simulink model "plant_2015B"  (R2015b)
settings: Solver=ode1  StartTime=0.0  StopTime=sim_time  FixedStep=0.001  RelTol=1e-3
undefined symbols (not defined in the file): Standard_Devices, UDP_Protocol, zh_step
libraries: sldrtlib x6, dspnetwork x2, powerlib_meascontrol x1
settings Model: Creator=Anony  LastModifiedBy=Anony

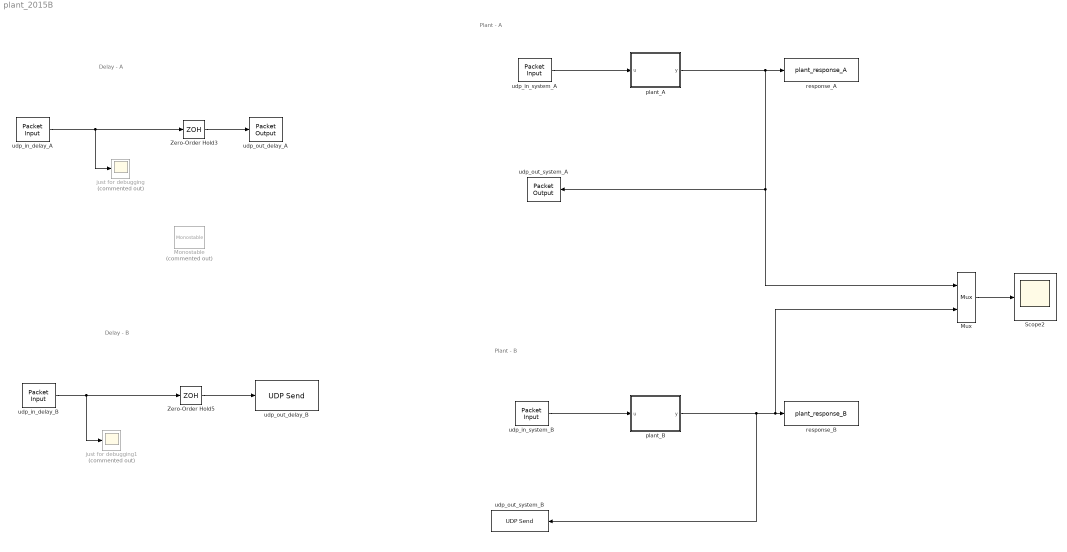
== system plant_2015B ==
  note: Plant - A
  note: Plant - B
  note: Delay - A
  note: Delay - B
  Monostable : powerlib_meascontrol/Logic/Monostable  Commented=on  EdgeDetect=Rising  PulseDuration=0.015  ic=0  Ts=0
  Mux : Mux  Inputs=2
  Scope2 : Scope
  Zero-Order Hold3 : ZeroOrderHold  SampleTime=zh_step
  Zero-Order Hold5 : ZeroOrderHold  SampleTime=zh_step
  just for debugging : Scope  Commented=on
  just for debugging1 : Scope  Commented=on
  plant_A : Subsystem
  plant_B : Subsystem
  response_A : ToWorkspace  VariableName=plant_response_A  SaveFormat=Timeseries  SampleTime=zh_step
  response_B : ToWorkspace  VariableName=plant_response_B  SaveFormat=Timeseries  SampleTime=zh_step
  udp_in_delay_A : sldrtlib/Packet Input  SampleTime=0.001  MaxMissedTicks=inf  ShowMissedTicks=off  YieldWhenWaiting=off  DrvName=Standard_Devices/UDP_Protocol  DrvAddress=27000  DrvOptions=[2468394754 27000]  PacketSize=8  DataTypes='double'  ShowReady=off  ShowError=off  PacketID=1  ByteOrder=1  ShowTimestamp=off
      settings: AttributesFormatString=Standard Devices\nUDP Protocol [6978h]
  udp_in_delay_B : sldrtlib/Packet Input  SampleTime=0.001  MaxMissedTicks=inf  ShowMissedTicks=off  YieldWhenWaiting=off  DrvName=Standard_Devices/UDP_Protocol  DrvAddress=27010  DrvOptions=[2468394754 27010]  PacketSize=8  DataTypes='double'  ShowReady=off  ShowError=off  PacketID=1  ByteOrder=1  ShowTimestamp=off
      settings: AttributesFormatString=Standard Devices\nUDP Protocol [6982h]
  udp_in_system_A : sldrtlib/Packet Input  SampleTime=0.001  MaxMissedTicks=inf  ShowMissedTicks=off  YieldWhenWaiting=off  DrvName=Standard_Devices/UDP_Protocol  DrvAddress=27500  DrvOptions=[2468394754 27500]  PacketSize=8  DataTypes='double'  ShowReady=off  ShowError=off  PacketID=1  ByteOrder=1  ShowTimestamp=off
      settings: AttributesFormatString=Standard Devices\nUDP Protocol [6B6Ch]
  udp_in_system_B : sldrtlib/Packet Input  SampleTime=0.001  MaxMissedTicks=inf  ShowMissedTicks=off  YieldWhenWaiting=off  DrvName=Standard_Devices/UDP_Protocol  DrvAddress=27510  DrvOptions=[2468394754 27510]  PacketSize=8  DataTypes='double'  ShowReady=off  ShowError=off  PacketID=1  ByteOrder=1  ShowTimestamp=off
      settings: AttributesFormatString=Standard Devices\nUDP Protocol [6B76h]
  udp_out_delay_A : sldrtlib/Packet Output  SampleTime=0.01  MaxMissedTicks=inf  ShowMissedTicks=off  YieldWhenWaiting=off  DrvName=Standard_Devices/UDP_Protocol  DrvAddress=28000  DrvOptions=[2468394754 28000]  PacketSize=8  DataTypes='double'  ShowReady=off  ShowError=off  PacketID=1  ByteOrder=1  InitialValue=[]  FinalValue=[]
      settings: AttributesFormatString=Standard Devices\nUDP Protocol [6D60h]
  udp_out_delay_B : dspnetwork/UDP Send  remoteURL='147.32.183.2'  remotePort=28010  localURL='0.0.0.0'  localPortSource=Automatically determine  localPort=27000  sampletime=-1  separateLengthPort=0
  udp_out_system_A : sldrtlib/Packet Output  SampleTime=0.01  MaxMissedTicks=inf  ShowMissedTicks=off  YieldWhenWaiting=off  DrvName=Standard_Devices/UDP_Protocol  DrvAddress=28500  DrvOptions=[2468394754 28500]  PacketSize=8  DataTypes='double'  ShowReady=off  ShowError=off  PacketID=1  ByteOrder=1  InitialValue=[]  FinalValue=[]
      settings: AttributesFormatString=Standard Devices\nUDP Protocol [6F54h]
  udp_out_system_B : dspnetwork/UDP Send  remoteURL='147.32.183.2'  remotePort=28510  localURL='0.0.0.0'  localPortSource=Automatically determine  localPort=27000  sampletime=-1  separateLengthPort=0
  wires:
  plant_A/1(y) -> response_A/1, udp_out_system_A/1, Mux/1
  udp_in_system_A/1 -> plant_A/1(u)
  udp_in_system_B/1 -> plant_B/1(u)
  plant_B/1(y) -> Mux/2, response_B/1, udp_out_system_B/1
  udp_in_delay_A/1 -> just for debugging/1, Zero-Order Hold3/1
  Zero-Order Hold3/1 -> udp_out_delay_A/1
  udp_in_delay_B/1 -> just for debugging1/1, Zero-Order Hold5/1
  Zero-Order Hold5/1 -> udp_out_delay_B/1
  Mux/1 -> Scope2/1

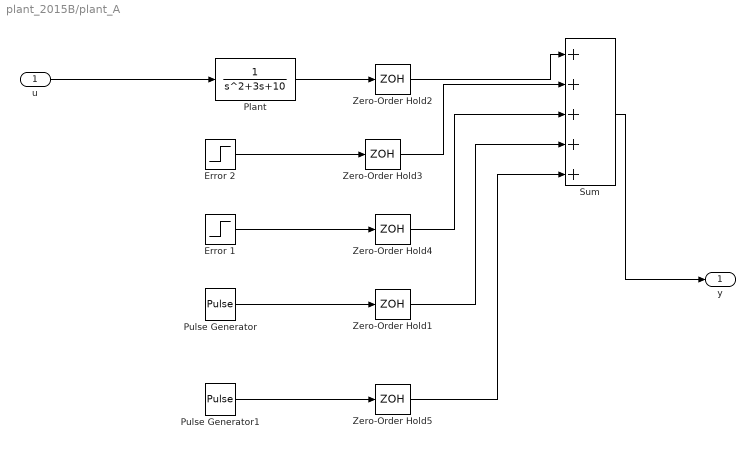
== system plant_2015B/plant_A ==
  u : Inport
  Error 1 : Step  Time=40  After=-0.4  SampleTime=0
  Error 2 : Step  Time=20  After=0.2  SampleTime=0
  Plant : TransferFcn  Denominator=[1 3 10]
  Pulse Generator : DiscretePulseGenerator  PulseType=Time based  Amplitude=0.3  Period=3  PulseWidth=5  PhaseDelay=15
  Pulse Generator1 : DiscretePulseGenerator  PulseType=Time based  Amplitude=-0.18  Period=3  PulseWidth=5  PhaseDelay=25
  Sum : Sum  Inputs=|+++++
  Zero-Order Hold{1..5} (5 alike) : ZeroOrderHold  SampleTime=zh_step
  y : Outport
  wires:
  Zero-Order Hold3/1 -> Sum/2
  Plant/1 -> Zero-Order Hold2/1
  Sum/1 -> y/1
  Zero-Order Hold2/1 -> Sum/1
  u/1 -> Plant/1
  Zero-Order Hold4/1 -> Sum/3
  Error 2/1 -> Zero-Order Hold3/1
  Error 1/1 -> Zero-Order Hold4/1
  Pulse Generator/1 -> Zero-Order Hold1/1
  Zero-Order Hold1/1 -> Sum/4
  Pulse Generator1/1 -> Zero-Order Hold5/1
  Zero-Order Hold5/1 -> Sum/5

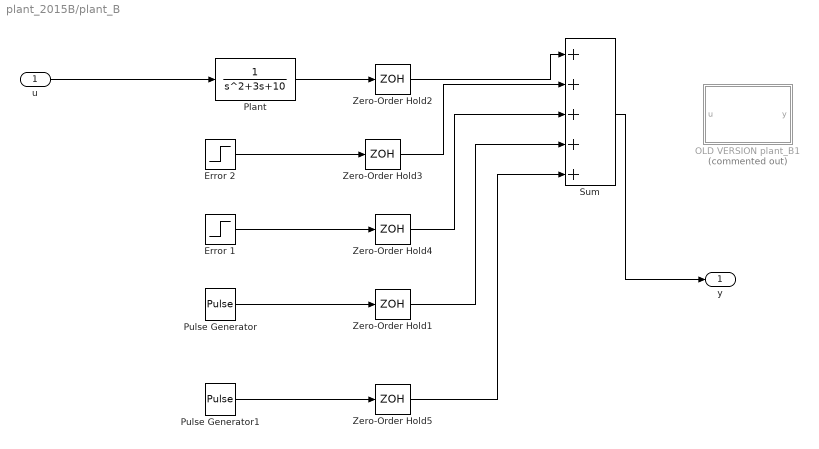
== system plant_2015B/plant_B ==
  u : Inport
  Error 1 : Step  Time=40  After=-0.4  SampleTime=0
  Error 2 : Step  Time=20  After=0.2  SampleTime=0
  OLD VERSION plant_B1 : Subsystem  Commented=on
  Plant : TransferFcn  Denominator=[1 3 10]
  Pulse Generator : DiscretePulseGenerator  PulseType=Time based  Amplitude=0.3  Period=3  PulseWidth=5  PhaseDelay=15
  Pulse Generator1 : DiscretePulseGenerator  PulseType=Time based  Amplitude=-0.18  Period=3  PulseWidth=5  PhaseDelay=25
  Sum : Sum  Inputs=|+++++
  Zero-Order Hold{1..5} (5 alike) : ZeroOrderHold  SampleTime=zh_step
  y : Outport
  wires:
  Zero-Order Hold5/1 -> Sum/5
  Pulse Generator1/1 -> Zero-Order Hold5/1
  Zero-Order Hold1/1 -> Sum/4
  Pulse Generator/1 -> Zero-Order Hold1/1
  Error 1/1 -> Zero-Order Hold4/1
  Error 2/1 -> Zero-Order Hold3/1
  Zero-Order Hold4/1 -> Sum/3
  u/1 -> Plant/1
  Zero-Order Hold2/1 -> Sum/1
  Sum/1 -> y/1
  Plant/1 -> Zero-Order Hold2/1
  Zero-Order Hold3/1 -> Sum/2

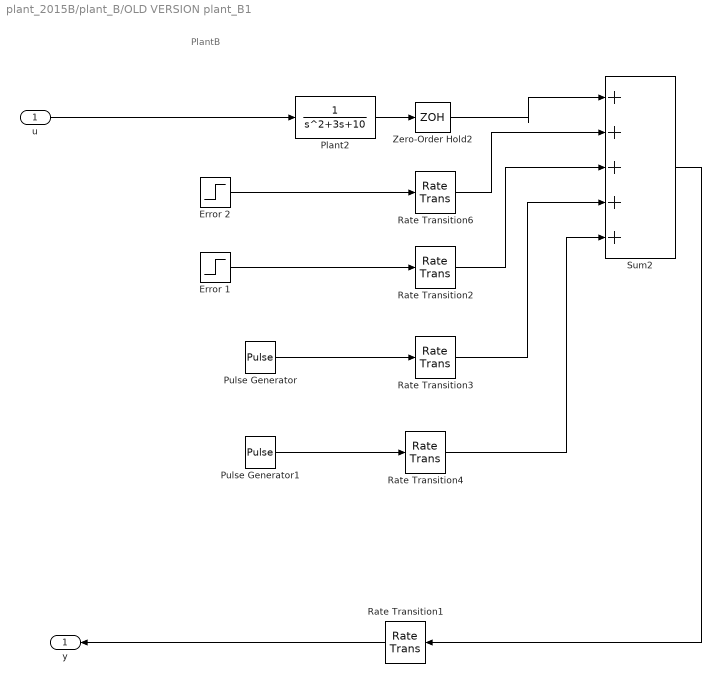
== system plant_2015B/plant_B/OLD VERSION plant_B1 ==
  note: PlantB
  u : Inport
  Error 1 : Step  Time=40  After=-0.4  SampleTime=0
  Error 2 : Step  Time=20  After=0.2  SampleTime=0
  Plant2 : TransferFcn  Denominator=[1 3 10]
  Pulse Generator : DiscretePulseGenerator  PulseType=Time based  Amplitude=0.3  Period=3  PulseWidth=5  PhaseDelay=15
  Pulse Generator1 : DiscretePulseGenerator  PulseType=Time based  Amplitude=-0.18  Period=3  PulseWidth=5  PhaseDelay=25
  Rate Transition1 : RateTransition  OutPortSampleTimeOpt=Inherit
  Rate Transition{2..4,6} (4 alike) : RateTransition  OutPortSampleTime=0.001
  Sum2 : Sum  Inputs=|+++++
  Zero-Order Hold2 : ZeroOrderHold  SampleTime=0.001
  y : Outport
  wires:
  Rate Transition4/1 -> Sum2/5
  Pulse Generator1/1 -> Rate Transition4/1
  Rate Transition3/1 -> Sum2/4
  Pulse Generator/1 -> Rate Transition3/1
  Zero-Order Hold2/1 -> Sum2/1
  Sum2/1 -> Rate Transition1/1
  Error 1/1 -> Rate Transition2/1
  Rate Transition1/1 -> y/1
  Rate Transition2/1 -> Sum2/3
  Rate Transition6/1 -> Sum2/2
  Plant2/1 -> Zero-Order Hold2/1
  Error 2/1 -> Rate Transition6/1
  u/1 -> Plant2/1
